simulink model "Fromworkspace"  (R2012b)
settings: Solver=ode45  StartTime=0.0  StopTime=5  RelTol=1e-3
libraries: opclib x5
settings Model: Creator=Josias  LastModifiedBy=Josias

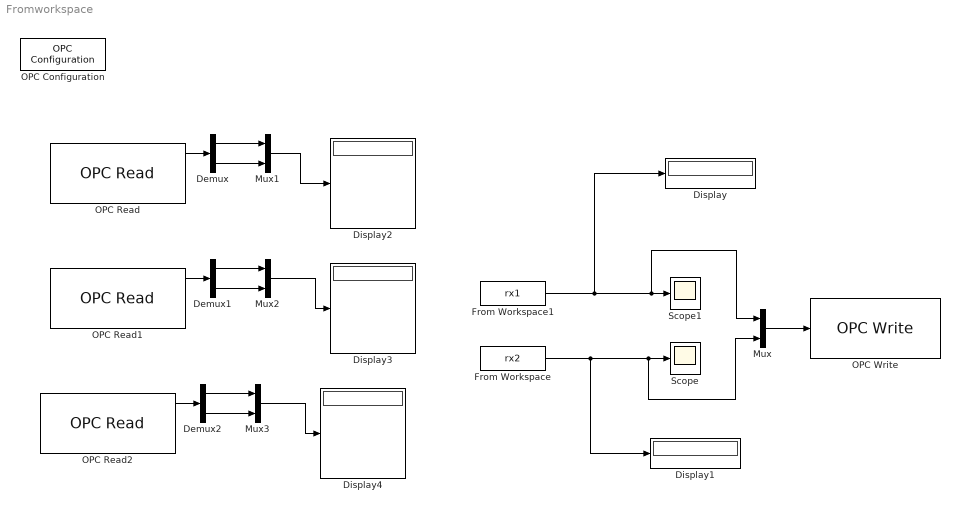
== system Fromworkspace ==
  Demux : Demux  Outputs=2
  Demux1 : Demux  Outputs=2
  Demux2 : Demux  Outputs=2
  Display{,1..4} (5 alike) : Display
  From Workspace : FromWorkspace  VariableName=rx2  SampleTime=0
  From Workspace1 : FromWorkspace  VariableName=rx1  SampleTime=0
  Mux{,1..3} (4 alike) : Mux  Inputs=2
  OPC Configuration : opclib/OPC Configuration  opcServers=localhost/ElipseSCADA.OPCSvr.1/10  errMissingItems=Error  errReadWrite=Warn  errShutdown=Error  errRTViolation=Warn  rtEnable=on  speedup=1  showLatency=off  beingUsed=on
  OPC Read : opclib/OPC Read  serverHost=localhost  serverID=ElipseSCADA.OPCSvr.1  itemIDs=Tags.Posição2, Tags.posição1  readMode=Synchronous (cache)  dataType=double  updateRate=0.5  showQual=on  showTS=on  tsMode=Seconds since start
  OPC Read1 : opclib/OPC Read  serverHost=localhost  serverID=ElipseSCADA.OPCSvr.1  itemIDs=Tags.sinal_junta_1, Tags.sinal_junta_2  readMode=Synchronous (cache)  dataType=double  updateRate=0.5  showQual=on  showTS=on  tsMode=Seconds since start
  OPC Read2 : opclib/OPC Read  serverHost=localhost  serverID=ElipseSCADA.OPCSvr.1  itemIDs=Tags.Erro_J1, Tags.Erro_J2  readMode=Synchronous (cache)  dataType=double  updateRate=0.5  showQual=on  showTS=on  tsMode=Seconds since start
  OPC Write : opclib/OPC Write  serverHost=localhost  serverID=ElipseSCADA.OPCSvr.1  itemIDs=Tags.setpoint_teta_1, Tags.setpoint_teta_2  writeMode=Synchronous  updateRate=0
  Scope : Scope
  Scope1 : Scope
      settings: TimeRange=10
  wires:
  From Workspace1/1 -> Display/1, Mux/1, Scope1/1
  From Workspace/1 -> Display1/1, Mux/2, Scope/1
  Mux/1 -> OPC Write/1
  OPC Read/1 -> Demux/1
  Demux/1 -> Mux1/1
  Demux/2 -> Mux1/2
  Mux1/1 -> Display2/1
  OPC Read1/1 -> Demux1/1
  Demux1/1 -> Mux2/1
  Demux1/2 -> Mux2/2
  Mux2/1 -> Display3/1
  OPC Read2/1 -> Demux2/1
  Demux2/1 -> Mux3/1
  Demux2/2 -> Mux3/2
  Mux3/1 -> Display4/1
